simulink model "SIMControlleurMAT"  (R2015a)
settings: Solver=ode45  StartTime=0.0  StopTime=50  RelTol=1e-3
settings Model: Creator=Utilisateur-pc  LastModifiedBy=ironi
settings DataIOCC: SignalLoggingSaveFormat=ModelDataLogs
settings OptimizationCC: ExpressionDepthLimit=2147483647
settings DebuggingCC: UnderspecifiedInitializationDetection=Classic  MergeDetectMultiDrivingBlocksExec=none  SolverPrmCheckMsg=warning  FcnCallInpInsideContextMsg=EnableAllAsWarning  StateNameClashWarn=warning
settings GRTTargetCC: CombineOutputUpdateFcns=off  GRTInterface=on

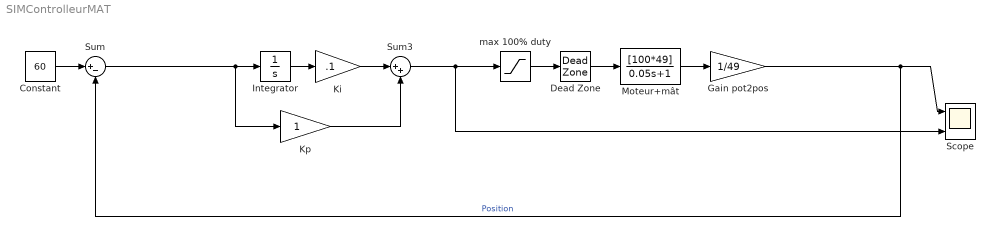
== system SIMControlleurMAT ==
  Constant : Constant  Value=60
  "Dead Zone " : DeadZone  LowerValue=-0.1  UpperValue=0.1  SaturateOnIntegerOverflow=on
  Gain pot2pos : Gain  Gain=1/49
  Integrator : Integrator
  Ki : Gain  Gain=.1
  Kp : Gain
  Moteur+mât : TransferFcn  Numerator=[100*49]  Denominator=[0.05 1]
  Scope : Scope  NumInputPorts=2
      settings: YMin=-5~-5  YMax=5~5
  Sum : Sum  Inputs=|+-  SampleTime=0.1
  Sum3 : Sum  Inputs=|++
  max 100% duty : Saturate  UpperLimit=12  LowerLimit=-12
  wires:
  Moteur+mât/1 -> Gain pot2pos/1
  Gain pot2pos/1 -> Scope/1, Sum/2  "Position"
  Constant/1 -> Sum/1
  max 100% duty/1 -> "Dead Zone "/1
  "Dead Zone "/1 -> Moteur+mât/1
  Sum/1 -> Integrator/1, Kp/1
  Integrator/1 -> Ki/1
  Sum3/1 -> max 100% duty/1, Scope/2
  Kp/1 -> Sum3/2
  Ki/1 -> Sum3/1
